simulink model "blobanalysis"  (R2020b)
settings: Solver=VariableStepAuto  StartTime=0.0  StopTime=10.0  RelTol=1e-3
model workspace (MAT data in the model file):
  BWSlices.slice_1 = [0 0 0 0 0 0 0 0 0 0 0 0 ... (24025 elements, 155x155)]
  BWSlices.slice_2 = [0 0 0 0 0 0 0 0 0 0 0 0 ... (24025 elements, 155x155)]
  BWSlices.slice_3 = [0 0 0 0 0 0 0 0 0 0 0 0 ... (24025 elements, 155x155)]
  BWSlices.slice_4 = [0 0 0 0 0 0 0 0 0 0 0 0 ... (24025 elements, 155x155)]
  BWSlices.slice_5 = [0 0 0 0 0 0 0 0 0 0 0 0 ... (24025 elements, 155x155)]
  BWSlices.slice_6 = [0 0 0 0 0 0 0 0 0 0 0 0 ... (24025 elements, 155x155)]
  BWSlices.slice_7 = [0 0 0 0 0 0 0 0 0 0 0 0 ... (24025 elements, 155x155)]
  BWSlices.slice_8 = [0 0 0 0 0 0 0 0 0 0 0 0 ... (24025 elements, 155x155)]
  BWSlices.slice_9 = [0 0 0 0 0 0 0 0 0 0 0 0 ... (24025 elements, 155x155)]
  BWSlices.slice_10 = [0 0 0 0 0 0 0 0 0 0 0 0 ... (24025 elements, 155x155)]
  BWSlices.slice_11 = [0 0 0 0 0 0 0 0 0 0 0 0 ... (24025 elements, 155x155)]
  BWSlices.slice_12 = [0 0 0 0 0 0 0 0 0 0 0 0 ... (24025 elements, 155x155)]
  BWSlices.slice_13 = [0 0 0 0 0 0 0 0 0 0 0 0 ... (24025 elements, 155x155)]
  BWSlices.slice_14 = [0 0 0 0 0 0 0 0 0 0 0 0 ... (24025 elements, 155x155)]
  BWSlices.slice_15 = [0 0 0 0 0 0 0 0 0 0 0 0 ... (24025 elements, 155x155)]
  BWSlices.slice_16 = [0 0 0 0 0 0 0 0 0 0 0 0 ... (24025 elements, 155x155)]
  BWSlices.slice_17 = [0 0 0 0 0 0 0 0 0 0 0 0 ... (24025 elements, 155x155)]
  BWSlices.slice_18 = [0 0 0 0 0 0 0 0 0 0 0 0 ... (24025 elements, 155x155)]
  BWSlices.slice_19 = [0 0 0 0 0 0 0 0 0 0 0 0 ... (24025 elements, 155x155)]
  BWSlices.slice_20 = [0 0 0 0 0 0 0 0 0 0 0 0 ... (24025 elements, 155x155)]
  BWSlices.slice_21 = [0 0 0 0 0 0 0 0 0 0 0 0 ... (24025 elements, 155x155)]
  BWSlices.slice_22 = [0 0 0 0 0 0 0 0 0 0 0 0 ... (24025 elements, 155x155)]
  BWSlices.slice_23 = [0 0 0 0 0 0 0 0 0 0 0 0 ... (24025 elements, 155x155)]
  BWSlices.slice_24 = [0 0 0 0 0 0 0 0 0 0 0 0 ... (24025 elements, 155x155)]
  BWSlices.slice_25 = [0 0 0 0 0 0 0 0 0 0 0 0 ... (24025 elements, 155x155)]
  BWSlices.slice_26 = [0 0 0 0 0 0 0 0 0 0 0 0 ... (24025 elements, 155x155)]
  BWSlices.slice_27 = [0 0 0 0 0 0 0 0 0 0 0 0 ... (24025 elements, 155x155)]
  BWSlices.slice_28 = [0 0 0 0 0 0 0 0 0 0 0 0 ... (24025 elements, 155x155)]
  BWSlices.slice_29 = [0 0 0 0 0 0 0 0 0 0 0 0 ... (24025 elements, 155x155)]
  BWSlices.slice_30 = [0 0 0 0 0 0 0 0 0 0 0 0 ... (24025 elements, 155x155)]
  BWSlices.slice_31 = [0 0 0 0 0 0 0 0 0 0 0 0 ... (24025 elements, 155x155)]
  BWSlices.slice_32 = [0 0 0 0 0 0 0 0 0 0 0 0 ... (24025 elements, 155x155)]
  BWSlices.slice_33 = [0 0 0 0 0 0 0 0 0 0 0 0 ... (24025 elements, 155x155)]
  BWSlices.slice_34 = [0 0 0 0 0 0 0 0 0 0 0 0 ... (24025 elements, 155x155)]
  BWSlices.slice_35 = [0 0 0 0 0 0 0 0 0 0 0 0 ... (24025 elements, 155x155)]
  BWSlices.slice_36 = [0 0 0 0 0 0 0 0 0 0 0 0 ... (24025 elements, 155x155)]
  BWSlices.slice_37 = [0 0 0 0 0 0 0 0 0 0 0 0 ... (24025 elements, 155x155)]
  BWSlices.slice_38 = [0 0 0 0 0 0 0 0 0 0 0 0 ... (24025 elements, 155x155)]
  BWSlices.slice_39 = [0 0 0 0 0 0 0 0 0 0 0 0 ... (24025 elements, 155x155)]
  BWSlices.slice_40 = [0 0 0 0 0 0 0 0 0 0 0 0 ... (24025 elements, 155x155)]
  BWSlices.slice_41 = [0 0 0 0 0 0 0 0 0 0 0 0 ... (24025 elements, 155x155)]
  BWSlices.slice_42 = [0 0 0 0 0 0 0 0 0 0 0 0 ... (24025 elements, 155x155)]
  BWSlices.slice_43 = [0 0 0 0 0 0 0 0 0 0 0 0 ... (24025 elements, 155x155)]
  BWSlices.slice_44 = [0 0 0 0 0 0 0 0 0 0 0 0 ... (24025 elements, 155x155)]
  BWSlices.slice_45 = [0 0 0 0 0 0 0 0 0 0 0 0 ... (24025 elements, 155x155)]
  BWSlices.slice_46 = [0 0 0 0 0 0 0 0 0 0 0 0 ... (24025 elements, 155x155)]
  BWSlices.slice_47 = [0 0 0 0 0 0 0 0 0 0 0 0 ... (24025 elements, 155x155)]
  BWSlices.slice_48 = [0 0 0 0 0 0 0 0 0 0 0 0 ... (24025 elements, 155x155)]
  BWSlices.slice_49 = [0 0 0 0 0 0 0 0 0 0 0 0 ... (24025 elements, 155x155)]
  BWSlices.slice_50 = [0 0 0 0 0 0 0 0 0 0 0 0 ... (24025 elements, 155x155)]
  BWSlices.slice_51 = [0 0 0 0 0 0 0 0 0 0 0 0 ... (24025 elements, 155x155)]
  BWSlices.slice_52 = [0 0 0 0 0 0 0 0 0 0 0 0 ... (24025 elements, 155x155)]
  BWSlices.slice_53 = [0 0 0 0 0 0 0 0 0 0 0 0 ... (24025 elements, 155x155)]
  BWSlices.slice_54 = [0 0 0 0 0 0 0 0 0 0 0 0 ... (24025 elements, 155x155)]
  BWSlices.slice_55 = [0 0 0 0 0 0 0 0 0 0 0 0 ... (24025 elements, 155x155)]
  BWSlices.slice_56 = [0 0 0 0 0 0 0 0 0 0 0 0 ... (24025 elements, 155x155)]
  BWSlices.slice_57 = [0 0 0 0 0 0 0 0 0 0 0 0 ... (24025 elements, 155x155)]
  BWSlices.slice_58 = [0 0 0 0 0 0 0 0 0 0 0 0 ... (24025 elements, 155x155)]
  BWSlices.slice_59 = [0 0 0 0 0 0 0 0 0 0 0 0 ... (24025 elements, 155x155)]
  BWSlices.slice_60 = [0 0 0 0 0 0 0 0 0 0 0 0 ... (24025 elements, 155x155)]
  BWSlices.slice_61 = [0 0 0 0 0 0 0 0 0 0 0 0 ... (24025 elements, 155x155)]
  BWSlices.slice_62 = [0 0 0 0 0 0 0 0 0 0 0 0 ... (24025 elements, 155x155)]
  BWSlices.slice_63 = [0 0 0 0 0 0 0 0 0 0 0 0 ... (24025 elements, 155x155)]
  BWSlices.slice_64 = [0 0 0 0 0 0 0 0 0 0 0 0 ... (24025 elements, 155x155)]
  BWSlices.slice_65 = [0 0 0 0 0 0 0 0 0 0 0 0 ... (24025 elements, 155x155)]
  BWSlices.slice_66 = [0 0 0 0 0 0 0 0 0 0 0 0 ... (24025 elements, 155x155)]
  BWSlices.slice_67 = [0 0 0 0 0 0 0 0 0 0 0 0 ... (24025 elements, 155x155)]
  BWSlices.slice_68 = [0 0 0 0 0 0 0 0 0 0 0 0 ... (24025 elements, 155x155)]
  BWSlices.slice_69 = [0 0 0 0 0 0 0 0 0 0 0 0 ... (24025 elements, 155x155)]
  BWSlices.slice_70 = [0 0 0 0 0 0 0 0 0 0 0 0 ... (24025 elements, 155x155)]
  BWSlices.slice_71 = [0 0 0 0 0 0 0 0 0 0 0 0 ... (24025 elements, 155x155)]
  BWSlices.slice_72 = [0 0 0 0 0 0 0 0 0 0 0 0 ... (24025 elements, 155x155)]
  BWSlices.slice_73 = [0 0 0 0 0 0 0 0 0 0 0 0 ... (24025 elements, 155x155)]
  BWSlices.slice_74 = [0 0 0 0 0 0 0 0 0 0 0 0 ... (24025 elements, 155x155)]
  BWSlices.slice_75 = [0 0 0 0 0 0 0 0 0 0 0 0 ... (24025 elements, 155x155)]
  BWSlices.slice_76 = [0 0 0 0 0 0 0 0 0 0 0 0 ... (24025 elements, 155x155)]
  BWSlices.slice_77 = [0 0 0 0 0 0 0 0 0 0 0 0 ... (24025 elements, 155x155)]
  BWSlices.slice_78 = [0 0 0 0 0 0 0 0 0 0 0 0 ... (24025 elements, 155x155)]
  BWSlices.slice_79 = [0 0 0 0 0 0 0 0 0 0 0 0 ... (24025 elements, 155x155)]
  BWSlices.slice_80 = [0 0 0 0 0 0 0 0 0 0 0 0 ... (24025 elements, 155x155)]
  BWSlices.slice_81 = [0 0 0 0 0 0 0 0 0 0 0 0 ... (24025 elements, 155x155)]
  BWSlices.slice_82 = [0 0 0 0 0 0 0 0 0 0 0 0 ... (24025 elements, 155x155)]
  BWSlices.slice_83 = [0 0 0 0 0 0 0 0 0 0 0 0 ... (24025 elements, 155x155)]
  BWSlices.slice_84 = [0 0 0 0 0 0 0 0 0 0 0 0 ... (24025 elements, 155x155)]
  BWSlices.slice_85 = [0 0 0 0 0 0 0 0 0 0 0 0 ... (24025 elements, 155x155)]
  BWSlices.slice_86 = [0 0 0 0 0 0 0 0 0 0 0 0 ... (24025 elements, 155x155)]
  BWSlices.slice_87 = [0 0 0 0 0 0 0 0 0 0 0 0 ... (24025 elements, 155x155)]
  BWSlices.slice_88 = [0 0 0 0 0 0 0 0 0 0 0 0 ... (24025 elements, 155x155)]
  BWSlices.slice_89 = [0 0 0 0 0 0 0 0 0 0 0 0 ... (24025 elements, 155x155)]
  BWSlices.slice_90 = [0 0 0 0 0 0 0 0 0 0 0 0 ... (24025 elements, 155x155)]
  BWSlices.slice_91 = [0 0 0 0 0 0 0 0 0 0 0 0 ... (24025 elements, 155x155)]
  BWSlices.slice_92 = [0 0 0 0 0 0 0 0 0 0 0 0 ... (24025 elements, 155x155)]
  BWSlices.slice_93 = [0 0 0 0 0 0 0 0 0 0 0 0 ... (24025 elements, 155x155)]
  BWSlices.slice_94 = [0 0 0 0 0 0 0 0 0 0 0 0 ... (24025 elements, 155x155)]
  BWSlices.slice_95 = [0 0 0 0 0 0 0 0 0 0 0 0 ... (24025 elements, 155x155)]
  BWSlices.slice_96 = [0 0 0 0 0 0 0 0 0 0 0 0 ... (24025 elements, 155x155)]
  BWSlices.slice_97 = [0 0 0 0 0 0 0 0 0 0 0 0 ... (24025 elements, 155x155)]
  BWSlices.slice_98 = [0 0 0 0 0 0 0 0 0 0 0 0 ... (24025 elements, 155x155)]
  BWSlices.slice_99 = [0 0 0 0 0 0 0 0 0 0 0 0 ... (24025 elements, 155x155)]
  BWSlices.slice_100 = [0 0 0 0 0 0 0 0 0 0 0 0 ... (24025 elements, 155x155)]
  BWSlices.slice_101 = [0 0 0 0 0 0 0 0 0 0 0 0 ... (24025 elements, 155x155)]
  BWSlices.slice_102 = [0 0 0 0 0 0 0 0 0 0 0 0 ... (24025 elements, 155x155)]
  BWSlices.slice_103 = [0 0 0 0 0 0 0 0 0 0 0 0 ... (24025 elements, 155x155)]
  BWSlices.slice_104 = [0 0 0 0 0 0 0 0 0 0 0 0 ... (24025 elements, 155x155)]
  BWSlices.slice_105 = [0 0 0 0 0 0 0 0 0 0 0 0 ... (24025 elements, 155x155)]
  BWSlices.slice_106 = [0 0 0 0 0 0 0 0 0 0 0 0 ... (24025 elements, 155x155)]
  BWSlices.slice_107 = [0 0 0 0 0 0 0 0 0 0 0 0 ... (24025 elements, 155x155)]
  BWSlices.slice_108 = [0 0 0 0 0 0 0 0 0 0 0 0 ... (24025 elements, 155x155)]
  BWSlices.slice_109 = [0 0 0 0 0 0 0 0 0 0 0 0 ... (24025 elements, 155x155)]
  BWSlices.slice_110 = [0 0 0 0 0 0 0 0 0 0 0 0 ... (24025 elements, 155x155)]
  BWSlices.slice_111 = [0 0 0 0 0 0 0 0 0 0 0 0 ... (24025 elements, 155x155)]
  BWSlices.slice_112 = [0 0 0 0 0 0 0 0 0 0 0 0 ... (24025 elements, 155x155)]
  BWSlices.slice_113 = [0 0 0 0 0 0 0 0 0 0 0 0 ... (24025 elements, 155x155)]
  BWSlices.slice_114 = [0 0 0 0 0 0 0 0 0 0 0 0 ... (24025 elements, 155x155)]
  BWSlices.slice_115 = [0 0 0 0 0 0 0 0 0 0 0 0 ... (24025 elements, 155x155)]
  BWSlices.slice_116 = [0 0 0 0 0 0 0 0 0 0 0 0 ... (24025 elements, 155x155)]
  BWSlices.slice_117 = [0 0 0 0 0 0 0 0 0 0 0 0 ... (24025 elements, 155x155)]
  BWSlices.slice_118 = [0 0 0 0 0 0 0 0 0 0 0 0 ... (24025 elements, 155x155)]
  BWSlices.slice_119 = [0 0 0 0 0 0 0 0 0 0 0 0 ... (24025 elements, 155x155)]
  BWSlices.slice_120 = [0 0 0 0 0 0 0 0 0 0 0 0 ... (24025 elements, 155x155)]
  BWSlices.slice_121 = [0 0 0 0 0 0 0 0 0 0 0 0 ... (24025 elements, 155x155)]
  BWSlices.slice_122 = [0 0 0 0 0 0 0 0 0 0 0 0 ... (24025 elements, 155x155)]
  BWSlices.slice_123 = [0 0 0 0 0 0 0 0 0 0 0 0 ... (24025 elements, 155x155)]
  BWSlices.slice_124 = [0 0 0 0 0 0 0 0 0 0 0 0 ... (24025 elements, 155x155)]
  BWSlices.slice_125 = [0 0 0 0 0 0 0 0 0 0 0 0 ... (24025 elements, 155x155)]
  BWSlices.slice_126 = [0 0 0 0 0 0 0 0 0 0 0 0 ... (24025 elements, 155x155)]
  BWSlices.slice_127 = [0 0 0 0 0 0 0 0 0 0 0 0 ... (24025 elements, 155x155)]
  BWSlices.slice_128 = [0 0 0 0 0 0 0 0 0 0 0 0 ... (24025 elements, 155x155)]
  BWSlices.slice_129 = [0 0 0 0 0 0 0 0 0 0 0 0 ... (24025 elements, 155x155)]
  BWSlices.slice_130 = [0 0 0 0 0 0 0 0 0 0 0 0 ... (24025 elements, 155x155)]
  BWSlices.slice_131 = [0 0 0 0 0 0 0 0 0 0 0 0 ... (24025 elements, 155x155)]
  BWSlices.slice_132 = [0 0 0 0 0 0 0 0 0 0 0 0 ... (24025 elements, 155x155)]
  BWSlices.slice_133 = [0 0 0 0 0 0 0 0 0 0 0 0 ... (24025 elements, 155x155)]
  BWSlices.slice_134 = [0 0 0 0 0 0 0 0 0 0 0 0 ... (24025 elements, 155x155)]
  BWSlices.slice_135 = [0 0 0 0 0 0 0 0 0 0 0 0 ... (24025 elements, 155x155)]
  BWSlices.slice_136 = [0 0 0 0 0 0 0 0 0 0 0 0 ... (24025 elements, 155x155)]
  BWSlices.slice_137 = [0 0 0 0 0 0 0 0 0 0 0 0 ... (24025 elements, 155x155)]
  BWSlices.slice_138 = [0 0 0 0 0 0 0 0 0 0 0 0 ... (24025 elements, 155x155)]
  BWSlices.slice_139 = [0 0 0 0 0 0 0 0 0 0 0 0 ... (24025 elements, 155x155)]
  BWSlices.slice_140 = [0 0 0 0 0 0 0 0 0 0 0 0 ... (24025 elements, 155x155)]
  BWSlices.slice_141 = [0 0 0 0 0 0 0 0 0 0 0 0 ... (24025 elements, 155x155)]
  BWSlices.slice_142 = [0 0 0 0 0 0 0 0 0 0 0 0 ... (24025 elements, 155x155)]
  BWSlices.slice_143 = [0 0 0 0 0 0 0 0 0 0 0 0 ... (24025 elements, 155x155)]
  BWSlices.slice_144 = [0 0 0 0 0 0 0 0 0 0 0 0 ... (24025 elements, 155x155)]
  BWSlices.slice_145 = [0 0 0 0 0 0 0 0 0 0 0 0 ... (24025 elements, 155x155)]
  BWSlices.slice_146 = [0 0 0 0 0 0 0 0 0 0 0 0 ... (24025 elements, 155x155)]
  BWSlices.slice_147 = [0 0 0 0 0 0 0 0 0 0 0 0 ... (24025 elements, 155x155)]
  BWSlices.slice_148 = [0 0 0 0 0 0 0 0 0 0 0 0 ... (24025 elements, 155x155)]
  BWSlices.slice_149 = [0 0 0 0 0 0 0 0 0 0 0 0 ... (24025 elements, 155x155)]
  BWSlices.slice_150 = [0 0 0 0 0 0 0 0 0 0 0 0 ... (24025 elements, 155x155)]
  BWSlices.slice_151 = [0 0 0 0 0 0 0 0 0 0 0 0 ... (24025 elements, 155x155)]
  BWSlices.slice_152 = [0 0 0 0 0 0 0 0 0 0 0 0 ... (24025 elements, 155x155)]
  BWSlices.slice_153 = [0 0 0 0 0 0 0 0 0 0 0 0 ... (24025 elements, 155x155)]
  BWSlices.slice_154 = [0 0 0 0 0 0 0 0 0 0 0 0 ... (24025 elements, 155x155)]
  BWSlices.slice_155 = [0 0 0 0 0 0 0 0 0 0 0 0 ... (24025 elements, 155x155)]
  BWSlices.slice_156 = [0 0 0 0 0 0 0 0 0 0 0 0 ... (24025 elements, 155x155)]
  BWSlices.slice_157 = [0 0 0 0 0 0 0 0 0 0 0 0 ... (24025 elements, 155x155)]
  BWSlices.slice_158 = [0 0 0 0 0 0 0 0 0 0 0 0 ... (24025 elements, 155x155)]
  BWSlices.slice_159 = [0 0 0 0 0 0 0 0 0 0 0 0 ... (24025 elements, 155x155)]
  BWSlices.slice_160 = [0 0 0 0 0 0 0 0 0 0 0 0 ... (24025 elements, 155x155)]
  BWSlices.slice_161 = [0 0 0 0 0 0 0 0 0 0 0 0 ... (24025 elements, 155x155)]
  BWSlices.slice_162 = [0 0 0 0 0 0 0 0 0 0 0 0 ... (24025 elements, 155x155)]
  BWSlices.slice_163 = [0 0 0 0 0 0 0 0 0 0 0 0 ... (24025 elements, 155x155)]
  BWSlices.slice_164 = [0 0 0 0 0 0 0 0 0 0 0 0 ... (24025 elements, 155x155)]
  BWSlices.slice_165 = [0 0 0 0 0 0 0 0 0 0 0 0 ... (24025 elements, 155x155)]
  BWSlices.slice_166 = [0 0 0 0 0 0 0 0 0 0 0 0 ... (24025 elements, 155x155)]
  BWSlices.slice_167 = [0 0 0 0 0 0 0 0 0 0 0 0 ... (24025 elements, 155x155)]
  BWSlices.slice_168 = [0 0 0 0 0 0 0 0 0 0 0 0 ... (24025 elements, 155x155)]
  BWSlices.slice_169 = [0 0 0 0 0 0 0 0 0 0 0 0 ... (24025 elements, 155x155)]
  BWSlices.slice_170 = [0 0 0 0 0 0 0 0 0 0 0 0 ... (24025 elements, 155x155)]
  counter = '170'
  modelSlice = [0 0 0 0 0 0 0 0 0 0 0 0 ... (24025 elements, 155x155)]
libraries: visionstatistics x1, visionsources x1
settings Model: SimulationMode=rapid-accelerator  ParameterArgumentNames=modelSlice  OrderedModelArguments=off  Creator=The MathWorks, Inc.  LastModifiedBy=chira

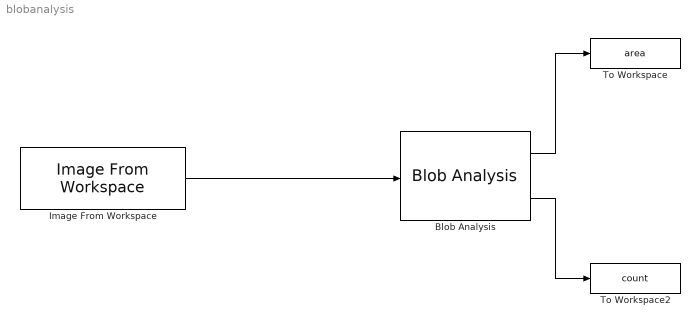
== system blobanalysis ==
  Blob Analysis : visionstatistics/Blob Analysis  Tag=vipblks_row_conv  area=on  centroid=off  bBox=off  majorAxis=off  minorAxis=off  angle=off  eccentricity=off  equivDiameterSq=off  extent=off  perimeter=off  outDT=double  conn=8  isLabel=off  maxBlobs=100  warnIfNumBlobsExceeded=off  isCount=on  useMinArea=off  minArea=0  useMaxArea=off  maxArea=intmax('uint32')  excludeBorderBlob=off  isOutVarDim=off  isFill=off  fillValues=-1  roundingMode=Floor  overflowMode=off  prodOutputMode=Binary point scaling  prodOutputWordLength=32  prodOutputFracLength=16  accumMode=Binary point scaling  accumWordLength=32  accumFracLength=0  firstCoeffMode=Binary point scaling  firstCoeffWordLength=16  firstCoeffFracLength=14  secondCoeffMode=Binary point scaling  secondCoeffWordLength=32  secondCoeffFracLength=16
      settings: SourceProductName=Computer Vision Toolbox
  Image From Workspace : visionsources/Image From Workspace  Tag=vipblks_nd  ImageValue=ImageValue  Ts=inf  imagePorts=One multidimensional signal  OutPortLabels=R|G|B  ImageDataType=boolean  Signed=on  WordLength=16  sdImageDataType=sfix(16)  FractionLengthMode=User-defined  FractionLength=15
      settings: SourceProductName=Computer Vision Toolbox
  To Workspace : ToWorkspace  VariableName=area  SaveFormat=Structure  SampleTime=-1
      settings: Save2DSignal=2-D array (concatenate along first dimension)
  To Workspace2 : ToWorkspace  VariableName=count  SampleTime=-1
      settings: Save2DSignal=2-D array (concatenate along first dimension)
  wires:
  Image From Workspace/1 -> Blob Analysis/1
  Blob Analysis/1 -> To Workspace/1
  Blob Analysis/2 -> To Workspace2/1
